simulink library "ground_visualization"  (R2016b)
settings: Solver=VariableStepAuto  StartTime=0.0  StopTime=10.0  RelTol=1e-3
undefined symbols (not defined in the file or in its folder): Earth, WGS84
libraries: aerolibtransform2 x1
settings Model: Creator=Sean  LastModifiedBy=Sean

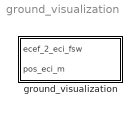
== system ground_visualization ==
  ground_visualization : Subsystem

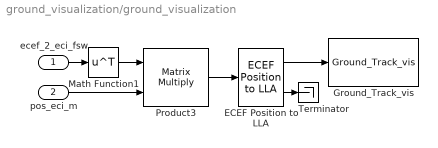
== system ground_visualization/ground_visualization ==
  ecef_2_eci_fsw : Inport
  pos_eci_m : Inport  Port=2
  ECEF Position to LLA : aerolibtransform2/ECEF Position to LLA  units=Metric (MKS)  ptype=Earth (WGS84)  F=1/298.257223563  R=6378137
  Ground_Track_vis : M-S-Function  FunctionName=Ground_Track_vis
  Math Function1 : Math  Operator=transpose  SaturateOnIntegerOverflow=on
  Product3 : Product  Multiplication=Matrix(*)
  Terminator : Terminator
  wires:
  Math Function1/1 -> Product3/1
  ecef_2_eci_fsw/1 -> Math Function1/1
  pos_eci_m/1 -> Product3/2
  Product3/1 -> ECEF Position to LLA/1
  ECEF Position to LLA/1 -> Ground_Track_vis/1
  ECEF Position to LLA/2 -> Terminator/1
